simulink model "compl"  (R2013a)
settings: Solver=FixedStepDiscrete  SolverMode=SingleTasking  StartTime=0.0  StopTime=inf  FixedStep=0.03  RelTol=1e-3
undefined symbols (not defined in the file): DiscIntNeverNeededParam
settings Model: SimulationMode=external  ExtModeTrigDuration=2  Creator=Alec  LastModifiedBy=user
settings OptimizationCC: ExpressionDepthLimit=2147483647  OptimizeModelRefInitCode=on  LifeSpan=1
settings DebuggingCC: SolverPrmCheckMsg=none  StrictBusMsg=Warning
settings HardwareCC: ProdBitPerInt=16  ProdBitPerPointer=8  ProdIntDivRoundTo=Zero  ProdEndianess=LittleEndian  ProdWordSize=8  ProdHWDeviceType=Atmel->AVR
settings RTWCC: SystemTargetFile=realtime.tlc  GenerateMakefile=off  TemplateMakefile=realtime.tmf  Description=Real-Time Toolbox  RTWVerbose=off  ProcessScript=realtime_make_rtw_hook
settings CodeAppCC: CustomSymbolStrType=$N$R$M  InternalIdentifier=Classic
settings STFCustomTargetCC: TargetLibSuffix=.a  GenerateSampleERTMain=on  ERTCustomFileBanners=on  SupportNonInlinedSFcns=off  SupportVariableSizeSignals=on  MATLABClassNameForMDSCustomization=Simulink.SoftwareTarget.ERTCustomization  SystemTargetFile=realtime.tlc
settings ERTTargetCC: ParMdlRefBuildCompliant=off  CompOptLevelCompliant=off  ConcurrentExecutionCompliant=off  CombineOutputUpdateFcns=off  ERTFirstTimeCompliant=off  SupportContinuousTime=on  SupportVariableSizeSignals=on  ModelStepFunctionPrototypeControlCompliant=off  CPPClassGenCompliant=off  ExtMode=on  ExtModeTransport=3  ExtModeMexFile=ext_serial_win32_comm  ExtModeMexArgs=0 12 115200  ERTSrcFileBannerTemplate=realtime_code_template.cgt  ERTHdrFileBannerTemplate=realtime_code_template.cgt  ERTDataSrcFileTemplate=realtime_code_template.cgt  ERTDataHdrFileTemplate=realtime_code_template.cgt  ERTCustomFileTemplate=realtime_file_process.tlc

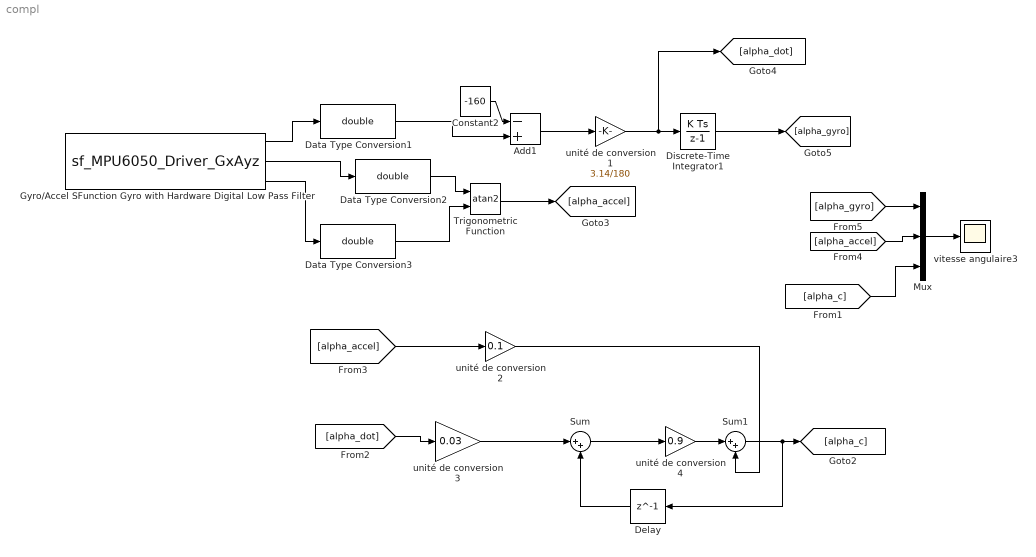
== system compl ==
  Add1 : Sum  Inputs=-+
  Constant2 : Constant  Value=-160
  Data Type Conversion1 : DataTypeConversion  OutDataTypeStr=double
  Data Type Conversion2 : DataTypeConversion  OutDataTypeStr=double
  Data Type Conversion3 : DataTypeConversion  OutDataTypeStr=double
  Delay : Delay  DelayLength=1
  Discrete-Time Integrator1 : DiscreteIntegrator  SampleTime=0.03  ICPrevOutput=DiscIntNeverNeededParam  ICPrevScaledInput=DiscIntNeverNeededParam
  Gyro/Accel SFunction Gyro with Hardware Digital Low Pass Filter : S-Function  InitFcn=try, set_param(gcb,'FunctionName','sf_MPU6050_Driver_GxAyz'), end  FunctionName=sf_MPU6050_Driver_GxAyz  SFunctionModules=sf_MPU6050_Driver_GxAyz_wrapper  EnableBusSupport=off  mask(S-Function Builder){}
      mask help: Simulink:masks:SFunctionBuilder_MD
      mask init:
      | val = [[.9  0.75 0.75 1 1 .9 .9 1]',[1 1 0.75 0.75 .9 .9 1 .9]'];try , sys = get_param(gcb,'SfunBuilderFcnName');if isempty(sys), sys = get_param(gcb,'FunctionName'); end,catch, sys = get_param(gcb,'FunctionName'); end
      settings: CopyFcn=set_param(gcbh,'LinkStatus','none')  PreSaveFcn=try, set_param(gcb,'FunctionName','sf_MPU6050_Driver_GxAyz'), end  OpenFcn=sfunctionwizard(gcbh)
      mask Display: plot(val(:,1),val(:,2)),disp(sys), port_label('output',1,'x_vel'), port_label('output',2,'y_acc'), port_label('output',3,'z_acc')
  Mux : Mux  Inputs=3
  Sum : Sum  Inputs=|++
  Sum1 : Sum  Inputs=|++
  Trigonometric Function : Trigonometry  Operator=atan2
  unité de conversion 1 : Gain  Gain=3.14/180
  unité de conversion 2 : Gain  Gain=0.1
  unité de conversion 3 : Gain  Gain=0.03
  unité de conversion 4 : Gain  Gain=0.9
  vitesse angulaire3 : Scope
      settings: TimeRange=10  YMin=3  YMax=18
  wires:
  unité de conversion 1/1 -> [alpha_dot], Discrete-Time Integrator1/1
  Discrete-Time Integrator1/1 -> [alpha_gyro]
  Gyro/Accel SFunction Gyro with Hardware Digital Low Pass Filter/1 -> Data Type Conversion1/1
  Gyro/Accel SFunction Gyro with Hardware Digital Low Pass Filter/2 -> Data Type Conversion2/1
  Gyro/Accel SFunction Gyro with Hardware Digital Low Pass Filter/3 -> Data Type Conversion3/1
  Data Type Conversion2/1 -> Trigonometric Function/1
  Data Type Conversion3/1 -> Trigonometric Function/2
  Trigonometric Function/1 -> [alpha_accel]
  Data Type Conversion1/1 -> Add1/2
  Constant2/1 -> Add1/1
  Add1/1 -> unité de conversion 1/1
  Mux/1 -> vitesse angulaire3/1
  [alpha_gyro] -> Mux/1
  [alpha_accel] -> Mux/2
  [alpha_accel] -> unité de conversion 2/1
  [alpha_dot] -> unité de conversion 3/1
  unité de conversion 3/1 -> Sum/1
  Sum/1 -> unité de conversion 4/1
  unité de conversion 4/1 -> Sum1/1
  Sum1/1 -> Delay/1, [alpha_c]
  Delay/1 -> Sum/2
  unité de conversion 2/1 -> Sum1/2
  [alpha_c] -> Mux/3
